simulink model "whole_topology"  (R2025a)
settings: Solver=VariableStepAuto  StartTime=0.0  StopTime=0.5  RelTol=1e-3
libraries: spsDiodeLib x7, spsVoltageMeasurementLib x4, spsACVoltageSourceLib x3, spsCurrentMeasurementLib x3, spsSeriesRLCBranchLib x3, spsDCMachineLib x1, spsDCVoltageSourceLib x1, spsIGBTLib x1, sps_lib x1
settings Model: Creator=yiğit  LastModifiedBy=yiğit

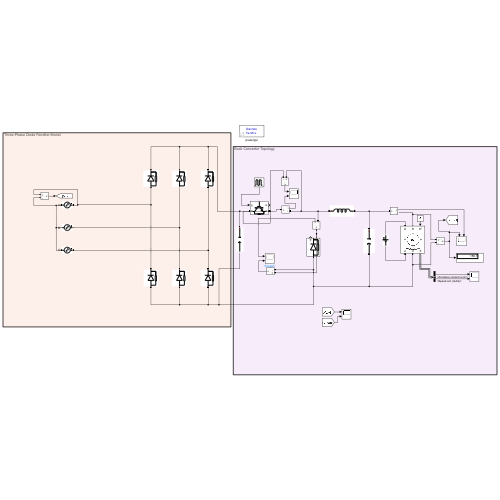
[thumbnail: Simulink's stored preview of the top-level diagram]
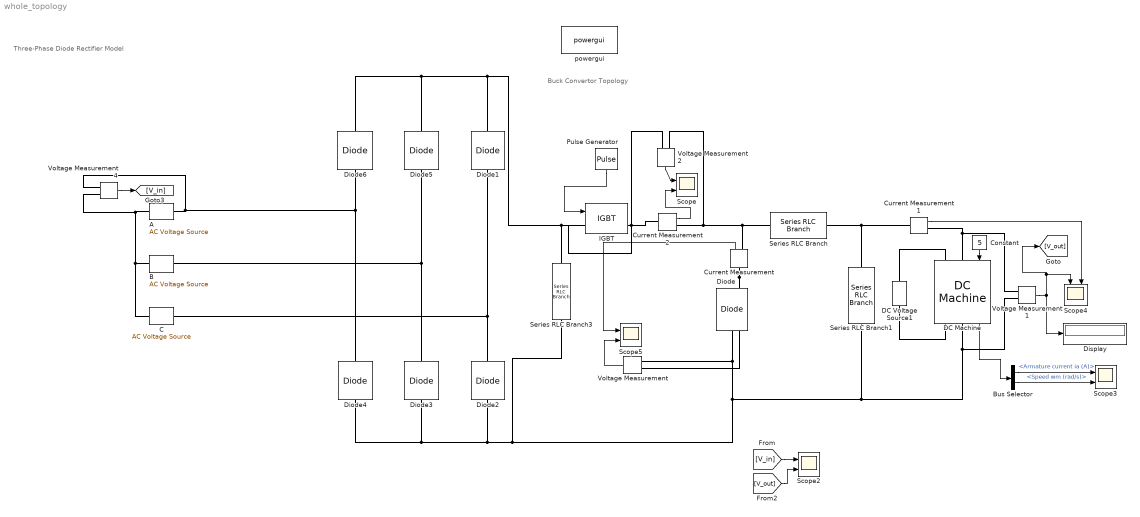
== system whole_topology ==
  note: Buck Convertor Topology
  note: Three-Phase Diode Rectifier Model
  A : spsACVoltageSourceLib/AC Voltage Source  Amplitude=136.082  Phase=0  Frequency=50  SampleTime=0  Measurements=None  BusType=swing  Pref=10e3  Qref=0  Qmin=-inf  Qmax=+inf
  B : spsACVoltageSourceLib/AC Voltage Source  Amplitude=136.082  Phase=120  Frequency=50  SampleTime=0  Measurements=None  BusType=swing  Pref=10e3  Qref=0  Qmin=-inf  Qmax=+inf
  Bus Selector : BusSelector  OutputSignals=Armature current ia (A),Speed wm (rad/s)
  C : spsACVoltageSourceLib/AC Voltage Source  Amplitude=136.082  Phase=240  Frequency=50  SampleTime=0  Measurements=None  BusType=swing  Pref=10e3  Qref=0  Qmin=-inf  Qmax=+inf
  Constant : Constant  Value=5
  Current Measurement : spsCurrentMeasurementLib/Current Measurement  PhasorSimulation=off  OutputType=Complex  PSBequivalent=0
  Current Measurement1 : spsCurrentMeasurementLib/Current Measurement  PhasorSimulation=off  OutputType=Complex  PSBequivalent=0
  Current Measurement2 : spsCurrentMeasurementLib/Current Measurement  PhasorSimulation=off  OutputType=Complex  PSBequivalent=0
  DC Machine : spsDCMachineLib/DC Machine  PresetModel=No  MechanicalLoad=Torque TL  FieldType=Wound  ShowDetailedParameters=on  MeasurementBus=off  RLa="[ 1.07  0.0245]"  RLf="[ 210  23]"  Laf=1.2  MachineConstant=Torque constant (N.m/A)  Ke=1.8  Kt=1.8  J=0.05  Bm=0  Tf=0  w0=1  Ifinit=1.04761904756944  TsPowergui=0  TsBlock=-1
  DC Voltage Source1 : spsDCVoltageSourceLib/DC Voltage Source  Amplitude=220  Measurements=None
  Diode : spsDiodeLib/Diode  Ron=0.001  Lon=0  Vf=0  IC=0  UseSnubber=0  Rs=1e6  Cs=1e-16  Measurements=on
  Diode{1..6} (6 alike) : spsDiodeLib/Diode  Ron=1e-3  Lon=0  Vf=0  IC=0  UseSnubber=0  Rs=1e6  Cs=1e-12  Measurements=off
  Display : Display
  IGBT : spsIGBTLib/IGBT  Ron=0.001  Lon=0  Vf=0  Tf=1e-6  Tt=2e-6  IC=0  Rs=1e5  Cs=inf  Measurements=on
  Pulse Generator : DiscretePulseGenerator  PulseType=Time based  Period=1e-3  PulseWidth=80
  Scope{,2..5} (5 alike) : Scope  NumInputPorts=2
      Scope settings: ActiveDisplayYMinimum=-386.69153856106936  ActiveDisplayYMaximum=162.16105918650862
      Scope2 settings: ActiveDisplayYMinimum=-201.45862541803965  ActiveDisplayYMaximum=452.30762876235713  YLabel=Voltage (V) and Current (A)  DataLoggingVariableName=ScopeData2
      Scope3 settings: ActiveDisplayYMinimum=-18.773978924329452  ActiveDisplayYMaximum=168.34562407576172  YLabel=Voltage (V) and Current (A)  DataLoggingVariableName=ScopeData3
      Scope4 settings: ActiveDisplayYMinimum=-60.369702307383207  ActiveDisplayYMaximum=342.02942694724663  YLabel=Voltage (V) and Current (A)  DataLoggingVariableName=ScopeData4
      Scope5 settings: ActiveDisplayYMinimum=-55.25741596096146  ActiveDisplayYMaximum=490.46354066565442  DataLoggingVariableName=ScopeData5
  Series RLC Branch : spsSeriesRLCBranchLib/Series RLC Branch  LConnTagsString=__new0  RConnTagsString=__new0  BranchType=L  Resistance=1  Inductance=12.5e-3  SetiL0=off  InitialCurrent=0  Capacitance=1e-6  Setx0=off  InitialVoltage=0  Measurements=None
  Series RLC Branch1 : spsSeriesRLCBranchLib/Series RLC Branch  LConnTagsString=__new0  RConnTagsString=__new0  BranchType=C  Resistance=1  Inductance=1e-3  SetiL0=off  InitialCurrent=0  Capacitance=220e-6  Setx0=off  InitialVoltage=0  Measurements=None
  Series RLC Branch3 : spsSeriesRLCBranchLib/Series RLC Branch  LConnTagsString=__new0  RConnTagsString=__new0  BranchType=C  Resistance=1  Inductance=1e-3  SetiL0=off  InitialCurrent=0  Capacitance=100e-6  Setx0=off  InitialVoltage=0  Measurements=None
  Voltage Measurement{,1..2,4} (4 alike) : spsVoltageMeasurementLib/Voltage Measurement  PhasorSimulation=off  OutputType=Complex  PSBequivalent=0
  powergui : sps_lib/powergui  Priority=1  SimulationMode=Discrete  SampleTime=5e-6  frequency=60  Iterations=50  frequencyindice=0  Pbase=100e6  ErrMax=1e-4  UnitsV=kV  UnitsW=MW  buscounter=0  FunctionMessages=off  echomessages=off  EnableUseOfTLC=off  CurrentSourceSwitches=off  DisableSnubberDevices=off  DisableRonSwitches=off  DisableVfSwitches=off  DisplayEquations=off  AutomaticDiscreteSolvers=off  SolverType=Tustin/Backward Euler (TBE)  Interpol=off  ExternalGateDelay=off  methode=off  Ts=100  x0status=blocks  SPID=on  SwTol=0  HookPort=off  NonlinearTolerance=1e-4  nMaxIteration=100  ContinueOnMaxIteration=off  RestoreLinks=warning  ResistiveCurrentMeasurement=off  Frange=[0:2:500]  Ylog=off  Xlog=on  ShowGrid=off  save=off  variable=ZData  structure=0  ZoomFFT=off  StartTime=0.0  cycles=1  DisplayStyle=1  fundamental=60  FreqAxis=off  MaxFrequency=1000  frequencyindicesteady=1  RmsSteady=1  display=off
  wires:
  DC Machine/1 -> Bus Selector/1
  Voltage Measurement1/1 -> [V_out], Scope4/1, Display/1
  Bus Selector/2 -> Scope3/2  "<Speed wm (rad/s)>"
  Constant/1 -> DC Machine/1
  Bus Selector/1 -> Scope3/1  "<Armature current ia (A)>"
  Current Measurement1/1 -> Scope4/2
  Voltage Measurement4/1 -> [V_in]
  [V_in] -> Scope2/1
  [V_out] -> Scope2/2
  Pulse Generator/1 -> IGBT/1
  Voltage Measurement/1 -> Scope5/2
  Current Measurement/1 -> Scope5/1
  Voltage Measurement2/1 -> Scope/1
  Current Measurement2/1 -> Scope/2
  connections:
  Series RLC Branch/RConn1 -- Series RLC Branch1/LConn1 -- Current Measurement1/LConn1
  Series RLC Branch3/LConn1 -- Voltage Measurement2/LConn2 -- IGBT/LConn1 -- Diode6/RConn1 -- Diode5/RConn1 -- Diode1/RConn1
  Current Measurement1/RConn1 -- Voltage Measurement1/LConn1 -- DC Machine/LConn1
  DC Voltage Source1/RConn1 -- DC Machine/LConn2
  DC Voltage Source1/LConn1 -- DC Machine/RConn2
  B/LConn1 -- C/LConn1 -- Voltage Measurement4/LConn2 -- A/LConn1
  Diode5/LConn1 -- B/RConn1 -- Diode3/RConn1
  A/RConn1 -- Diode6/LConn1 -- Diode4/RConn1 -- Voltage Measurement4/LConn1
  Diode1/LConn1 -- C/RConn1 -- Diode2/RConn1
  Diode4/LConn1 -- Diode3/LConn1 -- Voltage Measurement/LConn2 -- Diode/LConn1 -- Series RLC Branch1/RConn1 -- DC Machine/RConn1 -- Voltage Measurement1/LConn2 -- Series RLC Branch3/RConn1 -- Diode2/LConn1
  Diode/RConn1 -- Voltage Measurement/LConn1 -- Current Measurement/LConn1
  Current Measurement/RConn1 -- Current Measurement2/RConn1 -- Voltage Measurement2/LConn1 -- Series RLC Branch/LConn1
  IGBT/RConn1 -- Current Measurement2/LConn1
